simulink model "TarfficLightChart"  (R2018b)
settings: Solver=FixedStepDiscrete  StartTime=0.0  StopTime=10.0  RelTol=1e-3
settings Model: Creator=Ahmed Soliman  LastModifiedBy=Ahmed Soliman
settings OptimizationCC: DefaultParameterBehavior=Inlined  EnhancedBackFolding=on  PassReuseOutputArgsAs=Individual arguments  OptimizeBlockOrder=speed  DifferentSizesBufferReuse=on  OptimizationCustomize=off
settings DebuggingCC: UnderspecifiedInitializationDetection=Classic  MergeDetectMultiDrivingBlocksExec=none  ParameterTunabilityLossMsg=error
settings ModelReferenceCC: PropagateSignalLabelsOutOfModel=off
settings SFSimCC: MATLABDynamicMemAlloc=off
settings RTWCC: SystemTargetFile=ert.tlc  GenCodeOnly=on  TemplateMakefile=ert_default_tmf  GenerateReport=on  IncludeHyperlinkInReport=on  LaunchReport=on  GenerateTraceInfo=on  GenerateTraceReport=on  GenerateTraceReportSl=on  GenerateTraceReportSf=on  GenerateTraceReportEml=on
settings CodeAppCC: ForceParamTrailComments=on  IgnoreCustomStorageClasses=off  OperatorAnnotations=on  SimulinkDataObjDesc=on  SFDataObjDesc=on  InsertBlockDesc=on
settings ERTTargetCC: TargetLangStandard=C99 (ISO)  GenerateSampleERTMain=on  InlinedParameterPlacement=NonHierarchical  ERTCustomFileTemplate=example_file_process.tlc

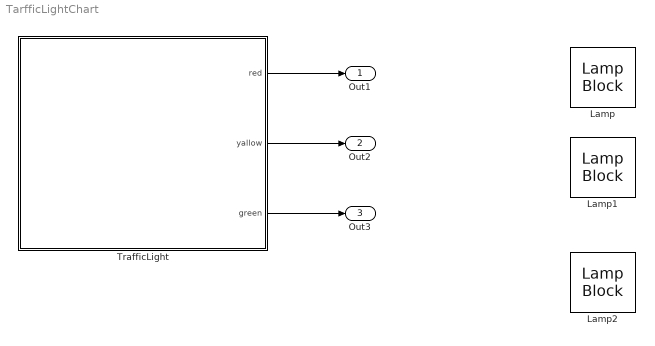
== system TarfficLightChart ==
  Lamp : LampBlock  WebBlockId=2
  Lamp1 : LampBlock  WebBlockId=3
  Lamp2 : LampBlock  WebBlockId=4
  TrafficLight : Stateflow chart  TreatAsAtomicUnit=on
  Out1 : Outport  OutDataTypeStr=uint8
  Out2 : Outport  Port=2  OutDataTypeStr=uint8
  Out3 : Outport  Port=3  OutDataTypeStr=uint8
  wires:
  TrafficLight/1(red) -> Out1/1
  TrafficLight/2(yallow) -> Out2/1
  TrafficLight/3(green) -> Out3/1

== stateflow chart TarfficLightChart/TrafficLight ==
  state Green
    en:
    red = 0;
    green = 1;
    yallow = 0;
    du:
    green = 1;
    ex:
  state Red
    en:
    red = 1;
    green = 0;
    yallow = 0;
    du:
    red = 1;
    ex:
  state Yallow
    en:
    red = 0;
    green = 0;
    yallow = 1;
    du:
    yallow = 1;
    ex:
  (default) -> Green
  Green -> Red : [after(3,sec)]
  Red -> Yallow : [after(3,sec)]
  Yallow -> Green : [after(3,sec)]
  data: red output uint8; yallow output uint8; green output uint8
